simulink model "analiseDiscreto"  (R2018a)
settings: Solver=ode1  StartTime=0.0  StopTime=Tsimu  FixedStep=p  RelTol=1e-3  EnableMultiTasking=on
values from neighbouring files (symbols this model uses):
  A = [(rgo*Cwro2 - Cwpg2) (rgo*Cwro3 - Cwpg3); (Cwro2 - Cwpo2) (Cwro3 - Cwpo3)]    [init.m]
  a0 = r0    (= 458.312763766)    [init.m]
  B = [1 0]'    [init.m]
  C = g/Aw*[1 1]    [init.m]
  f0 = 1/1000*2    (= 0.002)    [init.m]
  h = 1    [init.m]
  K0 = place(A, B, [-1 -0.002])    [init.m]
  N0 = 1/(C*inv(-1*(A - B*K0))*B)    [init.m]
  r0 = (rgo*Cwro4 - Cwpg4) - (rgo*Cwro3 - Cwpg3)*(Cwro4 - Cwpo4)/(Cwro3 - Cwpo3)    (= 458.312763766)    [init.m]
  Tsimu = 100e3    (= 100000)    [init.m]
  x0 = [-12 4]*0'    [init.m]
settings Model: Creator=alessandropeixoto  LastModifiedBy=Raposo
settings SolverCC: AutoInsertRateTranBlk=on
settings DataIOCC: LimitDataPoints=on
settings OptimizationCC: LifeSpan=inf
settings DebuggingCC: SFUnexpectedBacktrackingDiag=warning  SFNoUnconditionalDefaultTransitionDiag=warning  SFExecutionAtInitializationDiag=none
settings HardwareCC: ProdBitPerSizeT=32  ProdBitPerPtrDiffT=32  ProdWordSize=32  ProdHWDeviceType=Specified
settings ModelReferenceCC: PropagateSignalLabelsOutOfModel=off
settings CodeAppCC: StateflowObjectComments=on
settings GRTTargetCC: TargetLangStandard=C89/C90 (ANSI)
settings ConfigComp: CovMetricSettings=dw  CovHtmlReporting=on  CovSaveCumulativeToWorkspaceVar=on  CovSaveSingleToWorkspaceVar=on  CovExternalEMLEnable=off

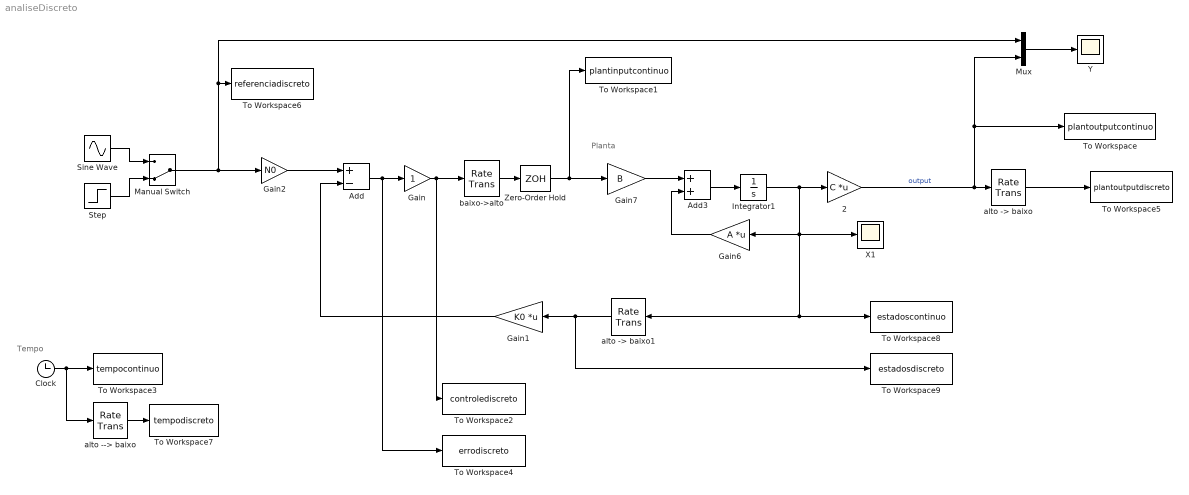
== system analiseDiscreto ==
  note: Tempo
  note: Planta
  " 2" : Gain  Gain=C  Multiplication=Matrix(K*u)
  Add : Sum  Inputs=+-
  Add3 : Sum
  Clock : Clock
  Gain : Gain
  Gain1 : Gain  Gain=K0  Multiplication=Matrix(K*u)
  Gain2 : Gain  Gain=N0
  Gain6 : Gain  Gain=A  Multiplication=Matrix(K*u)
  Gain7 : Gain  Gain=B
  Integrator1 : Integrator  InitialCondition=x0
  Manual Switch : ManualSwitch  CurrentSetting=0
  Mux : Mux  Inputs=2
  Sine Wave : Sin  Amplitude=a0  Frequency=f0  SampleTime=h
  Step : Step  Time=Tsimu/2  After=r0  SampleTime=0
  To Workspace : ToWorkspace  VariableName=plantoutputcontinuo  SampleTime=-1
  To Workspace1 : ToWorkspace  VariableName=plantinputcontinuo  SampleTime=-1
  To Workspace2 : ToWorkspace  VariableName=controlediscreto  SampleTime=h
  To Workspace3 : ToWorkspace  VariableName=tempocontinuo  SampleTime=-1
  To Workspace4 : ToWorkspace  VariableName=errodiscreto  SampleTime=h
  To Workspace5 : ToWorkspace  VariableName=plantoutputdiscreto  SampleTime=h
  To Workspace6 : ToWorkspace  VariableName=referenciadiscreto  SampleTime=h
  To Workspace7 : ToWorkspace  VariableName=tempodiscreto  SampleTime=h
  To Workspace8 : ToWorkspace  VariableName=estadoscontinuo  SampleTime=h
  To Workspace9 : ToWorkspace  VariableName=estadosdiscreto  SampleTime=h
  X1 : Scope
  Y : Scope
  Zero-Order Hold : ZeroOrderHold  SampleTime=-1
  alto --> baixo : RateTransition  OutPortSampleTime=h
  "alto -> baixo" : RateTransition  OutPortSampleTime=h
  "alto -> baixo1" : RateTransition  OutPortSampleTime=h
  baixo->alto : RateTransition
  wires:
  Gain/1 -> baixo->alto/1, To Workspace2/1
  Add/1 -> Gain/1, To Workspace4/1
  Clock/1 -> alto --> baixo/1, To Workspace3/1
  alto --> baixo/1 -> To Workspace7/1
  baixo->alto/1 -> Zero-Order Hold/1
  "alto -> baixo"/1 -> To Workspace5/1
  Gain1/1 -> Add/2
  Gain2/1 -> Add/1
  Sine Wave/1 -> Manual Switch/1
  Step/1 -> Manual Switch/2
  Manual Switch/1 -> Gain2/1, Mux/1, To Workspace6/1
  Gain7/1 -> Add3/1
  Add3/1 -> Integrator1/1
  Zero-Order Hold/1 -> To Workspace1/1, Gain7/1
  Integrator1/1 -> To Workspace8/1, "alto -> baixo1"/1, X1/1, Gain6/1, " 2"/1
  " 2"/1 -> Mux/2, To Workspace/1, "alto -> baixo"/1  "output"
  Gain6/1 -> Add3/2
  "alto -> baixo1"/1 -> To Workspace9/1, Gain1/1
  Mux/1 -> Y/1
